simulink model "cylindricalCell"  (R2022b)
settings: Solver=VariableStepAuto  StartTime=0.0  StopTime=10.0  RelTol=1e-3
libraries: fl_lib x2, moduleLibrary_lib x1, nesl_utility x1
settings Model: Creator=DELL  LastModifiedBy=DELL

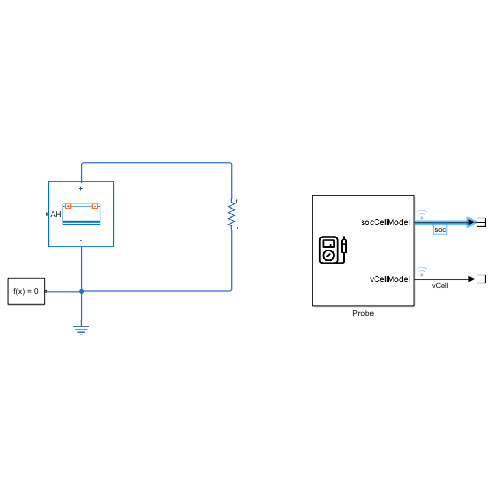
[thumbnail: Simulink's stored preview of the top-level diagram]
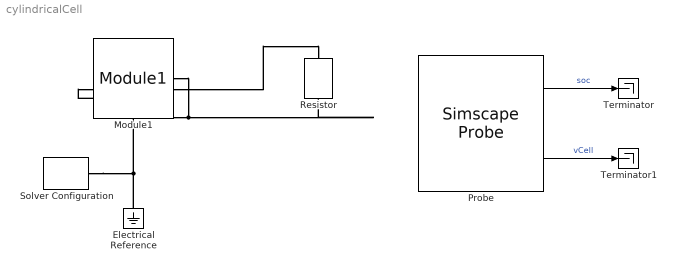
== system cylindricalCell ==
  Electrical Reference : fl_lib/Electrical/Electrical Elements/Electrical Reference
  Module1 : moduleLibrary_lib/Module1  SOC_vec=[0, .1, .25, .5, .75, .9, 1]  V0_vec=[3.5057, 3.566, 3.6337, 3.7127, 3.9259, 4.0777, 4.1928] V  V_range=[0, inf] V  R0_vec=[.0085, .0085, .0087, .0082, .0083, .0085, .0085] Ohm  AH=27 A*hr  extrapolation_option=simscape.enum.extrapolation.nearest  thermal_mass=100 J/K  AmbientResistance=25 K/W  P=4  S=13  SeriesGrouping=[1, 11, 1]  ParallelGrouping=[1, 1, 1]  iCellModel_specify=off  iCellModel_priority=None  iCellModel=repmat(0, 3, 1) A  iCellModel_nominal_specify=off  iCellModel_nominal_unit=A  iCellModel_nominal_value=1  vCellModel_specify=off  vCellModel_priority=None  vCellModel=repmat(0, 3, 1) V  vCellModel_nominal_specify=off  vCellModel_nominal_unit=V  vCellModel_nominal_value=1  socCellModel_specify=off  socCellModel_priority=High  socCellModel=repmat(1, 3, 1)  socCellModel_nominal_specify=off  socCellModel_nominal_unit=1  socCellModel_nominal_value=1  numCyclesCellModel_specify=off  numCyclesCellModel_priority=High  numCyclesCellModel=repmat(0, 3, 1)  numCyclesCellModel_nominal_specify=off  numCyclesCellModel_nominal_unit=1  numCyclesCellModel_nominal_value=1  temperatureCellModel_specify=off  temperatureCellModel_priority=High  temperatureCellModel=repmat(298.15, 3, 1) K  temperatureCellModel_nominal_specify=off  temperatureCellModel_nominal_unit=K  temperatureCellModel_nominal_value=1  vParallelAssembly_specify=off  vParallelAssembly_priority=None  vParallelAssembly=repmat(0, 13, 1) V  vParallelAssembly_nominal_specify=off  vParallelAssembly_nominal_unit=V  vParallelAssembly_nominal_value=1  socParallelAssembly_specify=off  socParallelAssembly_priority=None  socParallelAssembly=repmat(1, 13, 1)  socParallelAssembly_nominal_specify=off  socParallelAssembly_nominal_unit=1  socParallelAssembly_nominal_value=1
      settings: InternalSimscapePortConfiguration="{\"Bottom\":[{\"id\":\"n\",\"label\":\"-\",\"type\":\"foundation.electrical.electrical\"}],\"Left\":[{\"id\":\"AmbH\",\"label\":\"AH\",\"type\":\"foundation.thermal.thermal\"}],\"Right\":[],\"Top\":[{\"id\":\"p\",\"label\":\"+\",\"type\":\"foundation.electrical.electrical\"}]}"
  Probe : SimscapeProbe  BoundBlock=1  Variables={socCellModel, vCellModel}
  Resistor : fl_lib/Electrical/Electrical Elements/Resistor  R=1 Ohm  i_specify=off  i_priority=None  i=0 A  i_nominal_specify=off  i_nominal_unit=A  i_nominal_value=1  v_specify=off  v_priority=None  v=0 V  v_nominal_specify=off  v_nominal_unit=V  v_nominal_value=1
  Solver Configuration : nesl_utility/Solver Configuration  PhysicalDomain=network_engine_domain  SubClassName=solver  LeftPortType=input  RightPortType=generic  Tones=[]  Harmonics=[]  SimulateNoise=off  Profile=off  UseLocalSampling=off  EnableSwitchedLinearOptims=on  FrequencyDomain=off  UseCCode=off  RelTol=0.001  AbsTol=0.001  MinStep=1e-09  ToWorkspace=off  RevertToSquareIcSolve=off  NumHomotopyIterations=100  PhasorMode=off  PhasorModeNumHarmonics=1  ConsistencySolver=NEWTON_XTOL_AFTER_FTOL  IndexReductionMethod=DerivativeReplacement  DoDC=off  ResidualTolerance=1e-09  ConsistencyTolSource=GLOBAL  ConsistencyAbsTol=0.001  ConsistencyRelTol=0.001  ConsistencyTolFactor=0.001  UseLocalSolver=on  LocalSolverChoice=NE_BACKWARD_EULER_ADVANCER  ResolveIndetEquations=on  FunctionEvalNumThread=1  LocalSolverSampleTime=0.01  DoFixedCost=on  MaxNonlinIter=3  MaxModeIter=2  ComputeImpulses=off  ImpulseIterations=2  LinearAlgebra=auto  LinearAlgebraNumThread=0  EquationFormulation=NE_TIME_EF  DelaysMemoryBudget=1024  AutomaticFiltering=on  FilteringTimeConstant=0.001  PartitionStorageMethod=AS_NEEDED  PartitionMemoryBudget=1024  PartitionMethod=ROBUST
  Terminator : Terminator
  Terminator1 : Terminator
  wires:
  Probe/1 -> Terminator/1  "soc"
  Probe/2 -> Terminator1/1  "vCell"
  connections:
  Module1/LConn2 -- Resistor/LConn1
  Module1/RConn1 -- Solver Configuration/RConn1 -- Electrical Reference/LConn1 -- Resistor/RConn1
